simulink model "SimPowerSystems_PWM_Motor_4"  (R2014a)
settings: Solver=ode45  StartTime=0.0  StopTime=10  RelTol=1e-4
libraries: powerlib x4, powerlib_meascontrol x1
Description:
  | Copyright 2014 The MathWorks, Inc.
settings Model: Creator=smiller  LastModifiedBy=smiller
settings DataIOCC: SignalLoggingSaveFormat=ModelDataLogs
settings OptimizationCC: ExpressionDepthLimit=2147483647  InitFltsAndDblsToZero=on
settings DebuggingCC: SaveWithParameterizedLinksMsg=none  UnderspecifiedInitializationDetection=Classic  FcnCallInpInsideContextMsg=UseLocalSettings  StateNameClashWarn=warning
settings GRTTargetCC: TargetFcnLib=ansi_tfl_tmw.mat  CombineOutputUpdateFcns=off  GRTInterface=on

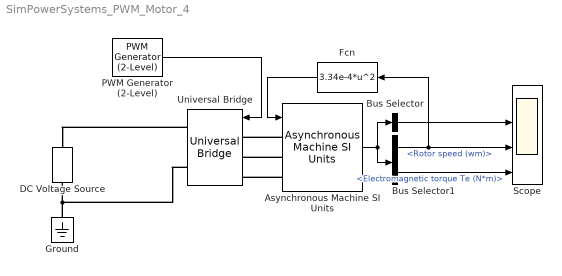
== system SimPowerSystems_PWM_Motor_4 ==
  Asynchronous Machine SI Units : powerlib/Machines/Asynchronous Machine SI Units  PresetModel=No  MechanicalLoad=Torque Tm  ShowDetailedParameters=on  RotorType=Squirrel-cage  ReferenceFrame=Rotor  Units=SI  MeasurementBus=off  NominalParameters=[3*746, 220, 60 ]  Stator=[1.115 0.005974]  Rotor=[1.083 0.005974]  Cage1=[ 0.022 0.226/377]  Cage2=[ 0.022 0.226/377]  Lm=0.2037  Mechanical=[0.02 0.005752 2]  PolePairs=2  InitialConditions=[1 0 0 0 0 0 0 0]  SimulateSaturation=off  Saturation=[14.03593122, 27.81365428, 53.79336849, 72.68890987, 97.98006896, 148.6815601, 215.7428561, 302.9841135, 420.4778367 ; 230, 322, 414, 460, 506, 552, 598, 644, 690]  LoadFlowParameters=1492000  TsPowergui=0  TsBlock=-1  IterativeModel=Trapezoidal non iterative  Pmec=0
  Bus Selector : BusSelector  OutputSignals=Stator measurements.Stator current is_a (A),Stator measurements.Stator current is_b (A),Stator measurements.Stator current is_c (A)  OutputAsBus=on
  Bus Selector1 : BusSelector  OutputSignals=Mechanical.Rotor speed (wm),Mechanical.Electromagnetic torque Te (N*m)
  DC Voltage Source : powerlib/Electrical Sources/DC Voltage Source  Amplitude=400  Measurements=None
  Fcn : Fcn  Expr=3.34e-4*u^2
  Ground : powerlib/Elements/Ground  LConnTagsString=a
  PWM Generator (2-Level) : powerlib_meascontrol/Pulse & Signal Generators/PWM Generator (2-Level)  ModulatorType=Three-phase bridge (6 pulses)  ModulatorMode=Unsynchronized  nF=27  Fc=18*60  ModulatingSignals=on  m=0.9  Freq=60  Phase=0  Ts=10e-6
  Scope : Scope  NumInputPorts=4
      settings: YMin=-5~-5~-5~-5  YMax=5~5~5~5
  Universal Bridge : powerlib/Power Electronics/Universal Bridge  Arms=3  SnubberResistance=1e5  SnubberCapacitance=inf  Device=IGBT / Diodes  Ron=1e-3  Lon=0  ForwardVoltages="[  0  0  ]"  ForwardVoltage=0  GTOparameters=[ 10e-6 , 20e-6 ]  IGBTparameters=[ 1e-6 , 1e-6 ]  Measurements=None  Measurements_2=None  converterType=Rectifier
  wires:
  PWM Generator (2-Level)/1 -> Universal Bridge/1
  Asynchronous Machine SI Units/1 -> Bus Selector/1, Bus Selector1/1
  Bus Selector/1 -> Scope/2
  Bus Selector1/1 -> Scope/3, Fcn/1  "<Rotor speed (wm)>"
  Bus Selector1/2 -> Scope/4  "<Electromagnetic torque Te (N*m)>"
  Fcn/1 -> Asynchronous Machine SI Units/1
  connections:
  Ground/LConn1 -- DC Voltage Source/LConn1 -- Universal Bridge/RConn2
  Universal Bridge/RConn1 -- DC Voltage Source/RConn1
  Asynchronous Machine SI Units/LConn1 -- Universal Bridge/LConn1
  Asynchronous Machine SI Units/LConn2 -- Universal Bridge/LConn2
  Asynchronous Machine SI Units/LConn3 -- Universal Bridge/LConn3
